simulink model "digital_loop"  (R2022b)
settings: Solver=VariableStepAuto  StartTime=0.0  StopTime=10.0  RelTol=1e-3
settings Model: Creator=amres  LastModifiedBy=amres

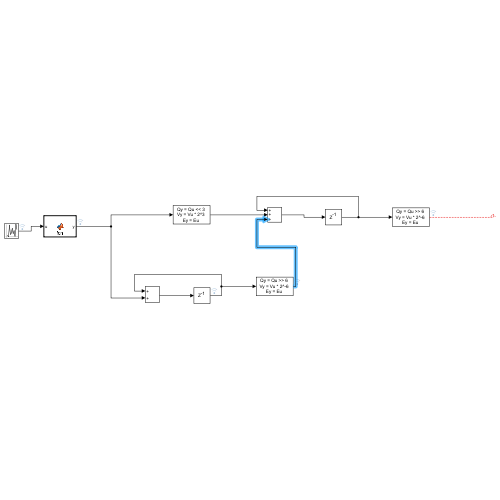
[thumbnail: Simulink's stored preview of the top-level diagram]
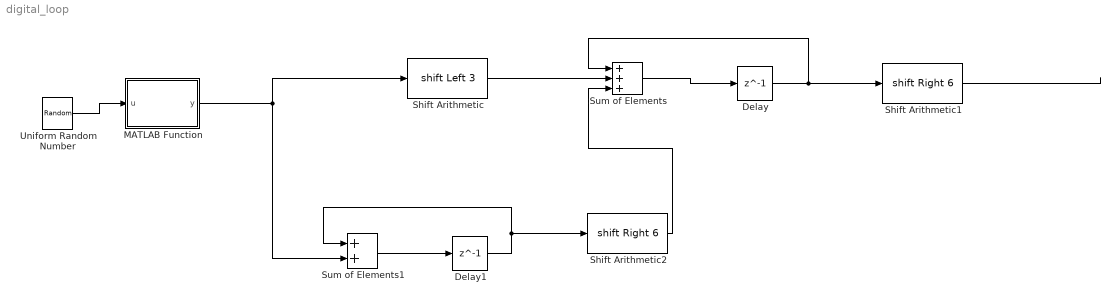
== system digital_loop ==
  Delay : Delay  DelayLength=1  InitialCondition=0  SampleTime=1
  Delay1 : Delay  DelayLength=1  InitialCondition=0  SampleTime=1
  MATLAB Function : MATLAB Function  TreatAsAtomicUnit=on
  Shift Arithmetic : ArithShift  BitShiftNumber=3  BitShiftDirection=Left
  Shift Arithmetic1 : ArithShift  BitShiftNumber=6  BitShiftDirection=Right
  Shift Arithmetic2 : ArithShift  BitShiftNumber=6  BitShiftDirection=Right
  Sum of Elements : Sum  Inputs=+++
  Sum of Elements1 : Sum
  Uniform Random Number : UniformRandomNumber  SampleTime=1
  wires:
  Delay/1 -> Shift Arithmetic1/1, Sum of Elements/1
  Shift Arithmetic/1 -> Sum of Elements/2
  Sum of Elements/1 -> Delay/1
  Shift Arithmetic2/1 -> Sum of Elements/3
  Sum of Elements1/1 -> Delay1/1
  MATLAB Function/1(y) -> Shift Arithmetic/1, Sum of Elements1/2
  Delay1/1 -> Sum of Elements1/1, Shift Arithmetic2/1
  Shift Arithmetic1/1 -> ?
  Uniform Random Number/1 -> MATLAB Function/1(u)

== matlab function digital_loop/MATLAB Function ==
  data: u input; y output
function y = fcn(u)
%#codegen
if u>0
    y=1;
else 
    y=-1;
end
